simulink model "R_SIPsim2022b"  (R2022b)
settings: Solver=ode45  StartTime=0.0  StopTime=50  FixedStep=0.01  RelTol=1e-3
values from neighbouring files (symbols this model uses):
  q0 = [0; pi/4; -pi/4]    [dynamics_without_simulink.m]    (also in final_simulation.m; simulation.m = zeros(3, 1))
  q0d = zeros(3, 1)    [dynamics_without_simulink.m]    (also in final_simulation.m; simulation.m)
settings Model: Creator=Utente  LastModifiedBy=danie
settings DebuggingCC: UnconnectedInputMsg=warning  UnconnectedOutputMsg=warning  UnconnectedLineMsg=warning
settings ModelReferenceCC: EnableRefExpFcnMdlSchedulingChecks=on
settings RTWCC: DLArmComputeVersion=19.05

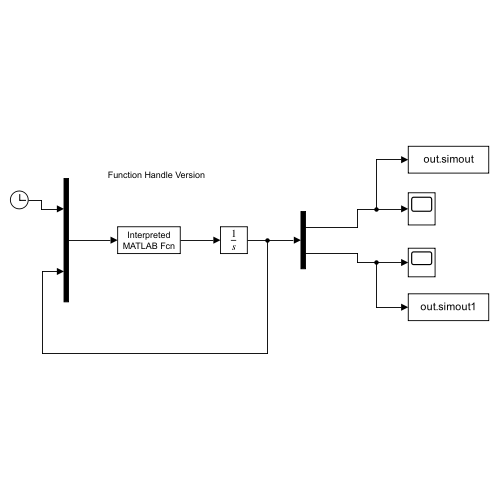
[thumbnail: Simulink's stored preview of the top-level diagram]
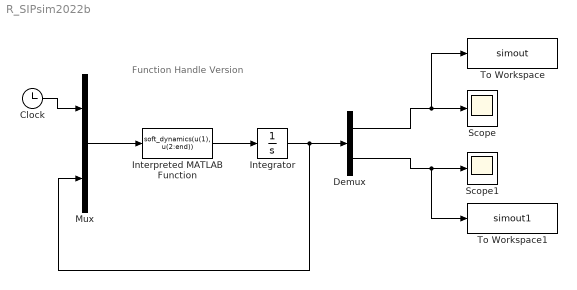
== system R_SIPsim2022b ==
  note: Function Handle Version
  Clock : Clock
  Demux : Demux  Outputs=2
  Integrator : Integrator  InitialCondition=[q0; q0d]
  Interpreted MATLAB Function : MATLABFcn  MATLABFcn=soft_dynamics(u(1), u(2:end))
  Mux : Mux  Inputs=2
  Scope : Scope
  Scope1 : Scope
  To Workspace : ToWorkspace  VariableName=simout  SaveFormat=Timeseries  SampleTime=-1
  To Workspace1 : ToWorkspace  VariableName=simout1  SaveFormat=Timeseries  SampleTime=-1
  wires:
  Mux/1 -> Interpreted MATLAB Function/1
  Clock/1 -> Mux/1
  Interpreted MATLAB Function/1 -> Integrator/1
  Integrator/1 -> Mux/2, Demux/1
  Demux/1 -> To Workspace/1, Scope/1
  Demux/2 -> To Workspace1/1, Scope1/1
